simulink model "motor_clarke_park_function_test_harness"  (R2023b)
settings: Solver=FixedStepDiscrete  StartTime=0.0  StopTime=0.001  FixedStep=0.001  RelTol=1e-3
settings Model: DataDictionary=motor_interface.sldd  Creator=user  LastModifiedBy=user

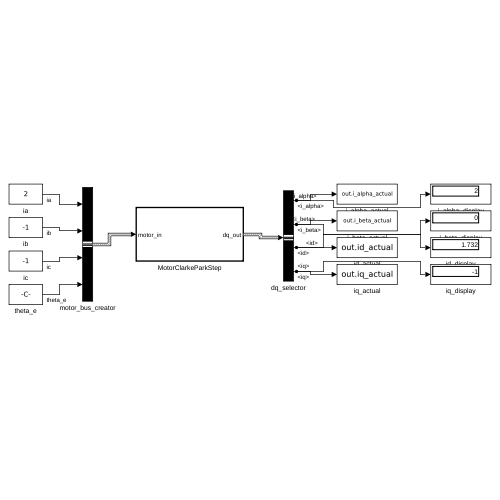
[thumbnail: Simulink's stored preview of the top-level diagram]
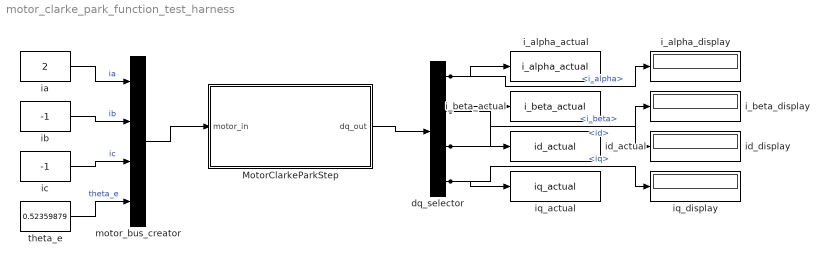
== system motor_clarke_park_function_test_harness ==
  MotorClarkeParkStep : Subsystem  TreatAsAtomicUnit=on  RTWFcnName=MotorClarkeParkStep  RTWFileName=MotorClarkeParkStep
      settings: RTWFcnNameOpts=User specified  RTWFileNameOpts=User specified
  dq_selector : BusSelector  OutputSignals=i_alpha,i_beta,id,iq
  i_alpha_actual : ToWorkspace  VariableName=i_alpha_actual  SaveFormat=Timeseries  SampleTime=-1
  i_alpha_display : Display
  i_beta_actual : ToWorkspace  VariableName=i_beta_actual  SaveFormat=Timeseries  SampleTime=-1
  i_beta_display : Display
  ia : Constant  Value=2  OutDataTypeStr=T_MotorCurrent  SampleTime=0.001
  ib : Constant  Value=-1  OutDataTypeStr=T_MotorCurrent  SampleTime=0.001
  ic : Constant  Value=-1  OutDataTypeStr=T_MotorCurrent  SampleTime=0.001
  id_actual : ToWorkspace  VariableName=id_actual  SaveFormat=Timeseries  SampleTime=-1
  id_display : Display
  iq_actual : ToWorkspace  VariableName=iq_actual  SaveFormat=Timeseries  SampleTime=-1
  iq_display : Display
  motor_bus_creator : BusCreator  Inputs=4  OutDataTypeStr=Bus: motor_t  NonVirtualBus=on
  theta_e : Constant  Value=0.52359879  OutDataTypeStr=T_MotorAngle  SampleTime=0.001
  wires:
  ia/1 -> motor_bus_creator/1  "ia"
  ib/1 -> motor_bus_creator/2  "ib"
  ic/1 -> motor_bus_creator/3  "ic"
  theta_e/1 -> motor_bus_creator/4  "theta_e"
  motor_bus_creator/1 -> MotorClarkeParkStep/1(motor_in)
  MotorClarkeParkStep/1(dq_out) -> dq_selector/1
  dq_selector/1 -> i_alpha_actual/1, i_alpha_display/1  "<i_alpha>"
  dq_selector/2 -> i_beta_actual/1, i_beta_display/1  "<i_beta>"
  dq_selector/3 -> id_actual/1, id_display/1  "<id>"
  dq_selector/4 -> iq_actual/1, iq_display/1  "<iq>"

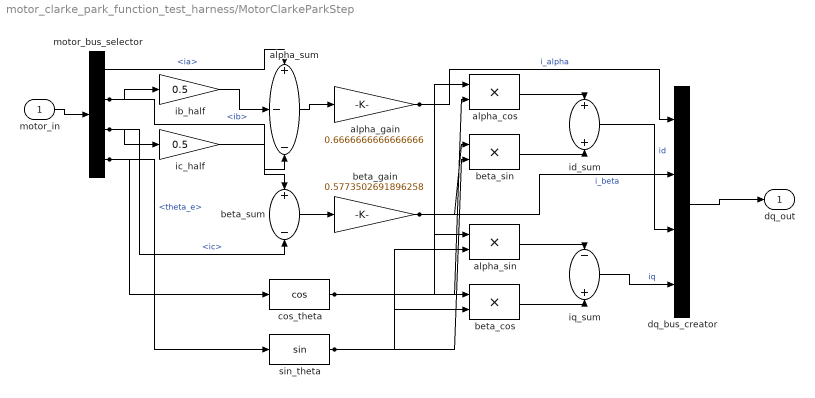
== system motor_clarke_park_function_test_harness/MotorClarkeParkStep ==
  motor_in : Inport  OutDataTypeStr=Bus: motor_t  BusOutputAsStruct=on
  alpha_cos : Product  Inputs=**  OutDataTypeStr=T_MotorCurrent  SaturateOnIntegerOverflow=on
  alpha_gain : Gain  Gain=0.6666666666666666  ParamDataTypeStr=T_MotorCurrent  OutDataTypeStr=T_MotorCurrent  SaturateOnIntegerOverflow=on
  alpha_sin : Product  Inputs=**  OutDataTypeStr=T_MotorCurrent  SaturateOnIntegerOverflow=on
  alpha_sum : Sum  Inputs=+--  OutDataTypeStr=T_MotorCurrent  AccumDataTypeStr=T_MotorCurrent  SaturateOnIntegerOverflow=on
  beta_cos : Product  Inputs=**  OutDataTypeStr=T_MotorCurrent  SaturateOnIntegerOverflow=on
  beta_gain : Gain  Gain=0.5773502691896258  ParamDataTypeStr=T_MotorCurrent  OutDataTypeStr=T_MotorCurrent  SaturateOnIntegerOverflow=on
  beta_sin : Product  Inputs=**  OutDataTypeStr=T_MotorCurrent  SaturateOnIntegerOverflow=on
  beta_sum : Sum  Inputs=+-  OutDataTypeStr=T_MotorCurrent  AccumDataTypeStr=T_MotorCurrent  SaturateOnIntegerOverflow=on
  cos_theta : Trigonometry  Operator=cos
  dq_bus_creator : BusCreator  Inputs=4  OutDataTypeStr=Bus: motor_dq_t  NonVirtualBus=on
  ib_half : Gain  Gain=0.5  ParamDataTypeStr=T_MotorCurrent  OutDataTypeStr=T_MotorCurrent  SaturateOnIntegerOverflow=on
  ic_half : Gain  Gain=0.5  ParamDataTypeStr=T_MotorCurrent  OutDataTypeStr=T_MotorCurrent  SaturateOnIntegerOverflow=on
  id_sum : Sum  OutDataTypeStr=T_MotorCurrent  AccumDataTypeStr=T_MotorCurrent  SaturateOnIntegerOverflow=on
  iq_sum : Sum  Inputs=-+  OutDataTypeStr=T_MotorCurrent  AccumDataTypeStr=T_MotorCurrent  SaturateOnIntegerOverflow=on
  motor_bus_selector : BusSelector  OutputSignals=ia,ib,ic,theta_e
  sin_theta : Trigonometry
  dq_out : Outport  OutDataTypeStr=Bus: motor_dq_t
  wires:
  dq_bus_creator/1 -> dq_out/1
  iq_sum/1 -> dq_bus_creator/4  "iq"
  id_sum/1 -> dq_bus_creator/3  "id"
  beta_cos/1 -> iq_sum/2
  alpha_sin/1 -> iq_sum/1
  beta_sin/1 -> id_sum/2
  alpha_cos/1 -> id_sum/1
  sin_theta/1 -> alpha_sin/2, beta_sin/2
  beta_gain/1 -> dq_bus_creator/2, beta_cos/1, beta_sin/1  "i_beta"
  cos_theta/1 -> beta_cos/2, alpha_cos/2
  alpha_gain/1 -> dq_bus_creator/1, alpha_sin/1, alpha_cos/1  "i_alpha"
  motor_bus_selector/4 -> sin_theta/1, cos_theta/1  "<theta_e>"
  beta_sum/1 -> beta_gain/1
  alpha_sum/1 -> alpha_gain/1
  ic_half/1 -> alpha_sum/3
  ib_half/1 -> alpha_sum/2
  motor_bus_selector/3 -> beta_sum/2, ic_half/1  "<ic>"
  motor_bus_selector/2 -> beta_sum/1, ib_half/1  "<ib>"
  motor_bus_selector/1 -> alpha_sum/1  "<ia>"
  motor_in/1 -> motor_bus_selector/1
